simulink model "PulseWidthCalculation"  (R2015b)
settings: Solver=FixedStepDiscrete  StartTime=0.0  StopTime=15  FixedStep=0.01  RelTol=1e-3
undefined symbols (not defined in the file): sigbuilder_block
libraries: simulink x2
settings Model: Creator=MELBAZ1  LastModifiedBy=MELBAZ1

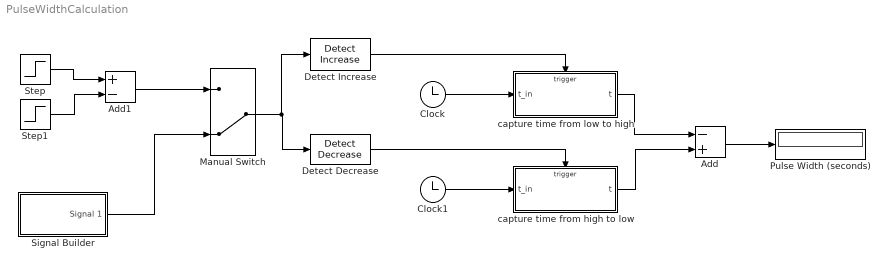
== system PulseWidthCalculation ==
  Add : Sum  Inputs=-+
  Add1 : Sum  Inputs=+-
  Clock : Clock
  Clock1 : Clock
  Detect Decrease : simulink/Logic and Bit Operations/Detect Decrease  vinit=0.0  InputProcessing=Inherited  OutDataTypeStr=boolean
  Detect Increase : simulink/Logic and Bit Operations/Detect Increase  vinit=0.0  InputProcessing=Inherited  OutDataTypeStr=boolean
  Manual Switch : ManualSwitch  CurrentSetting=0
  Pulse Width (seconds) : Display
  Signal Builder : Subsystem  Tag=STV Subsys  LoadFcn=sigbuilder_block('load');  StartFcn=sigbuilder_block('start');  StopFcn=sigbuilder_block('stop');  ClipboardFcn=sigbuilder_block('clipboard');  mask(Sigbuilder block){}
      mask help: Simulink:masks:SigbuilderBlock_MD
      mask init:
      | if ~strcmp(get_param(bdroot(gcbh),'SimulationStatus'),'stopped') tuvar = sigbuilder_block('maskInit'); end
      settings: CopyFcn=sigbuilder_block('copy');  DeleteFcn=sigbuilder_block('delete');  ModelCloseFcn=sigbuilder_block('modelClose');  PreSaveFcn=sigbuilder_block('preSave');  PauseFcn=sigbuilder_block('pause');  ContinueFcn=sigbuilder_block('continue');  NameChangeFcn=sigbuilder_block('namechange');  OpenFcn=sigbuilder_block('open',[453.6 124.2 550.8 400.2 ]);  CloseFcn=sigbuilder_block('close');
      mask Display: plot(0, 0, 100, 100,[2, 2, 32, 32, 2], [68, 8, 8, 68, 68],[32, 2], [38, 38], [32, 19, 2],[53, 60, 44], [32, 17, 17, 2],[16, 16, 31, 31]);txt = getActiveGroup(gcbh);text(2, 100, txt,'verticalAlignment', 'top');
  Step : Step  SampleTime=0.01
  Step1 : Step  Time=1.5  SampleTime=0.01
  capture time from high to low : Subsystem  TreatAsAtomicUnit=on
  "capture time from low to high " : Subsystem  TreatAsAtomicUnit=on
  wires:
  Detect Increase/1 -> "capture time from low to high "/Trigger
  Clock/1 -> "capture time from low to high "/1(t_in)
  Detect Decrease/1 -> capture time from high to low/Trigger
  "capture time from low to high "/1(t) -> Add/1
  capture time from high to low/1(t) -> Add/2
  Clock1/1 -> capture time from high to low/1(t_in)
  Add/1 -> Pulse Width (seconds)/1
  Step/1 -> Add1/1
  Step1/1 -> Add1/2
  Manual Switch/1 -> Detect Increase/1, Detect Decrease/1
  Add1/1 -> Manual Switch/1
  Signal Builder/1(Signal 1) -> Manual Switch/2

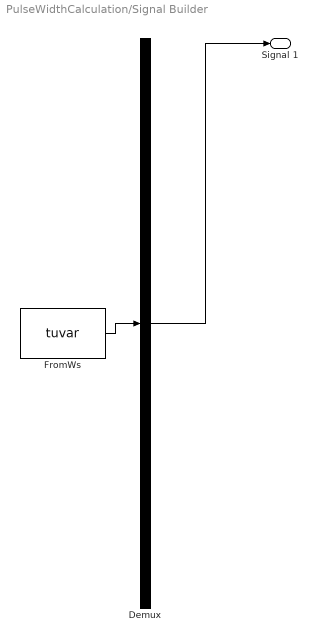
== system PulseWidthCalculation/Signal Builder ==
  Demux : Demux  Tag=STV Demux  Outputs=1
  FromWs : FromWorkspace  Tag=STV FromWs  VariableName=tuvar  SampleTime=0
      SigBuilderData=|
      | common.afterFinalStr = 'Extrapolate'
      | common.sampleTime = 0
      | dataSet.timeRange = [0 10]
      | dataSet.name = 'Group 1'
      | sbobj.Groups.Name = 'Group 1'
      | sbobj.Groups.Signals.Name = 'Signal 1'
      | sbobj.Groups.Signals.XData = [0 4 4 6 6 10]
      | sbobj.Groups.Signals.YData = [0 0 1 1 0 0]
  Signal 1 : Outport  Tag=STV Outport
  wires:
  Demux/1 -> Signal 1/1
  FromWs/1 -> Demux/1

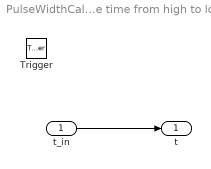
== system PulseWidthCalculation/capture time from high to low ==
  t_in : Inport
  Trigger : TriggerPort
  t : Outport
  wires:
  t_in/1 -> t/1

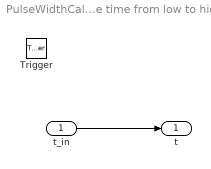
== system PulseWidthCalculation/capture time from low to high  ==
  t_in : Inport
  Trigger : TriggerPort
  t : Outport
  wires:
  t_in/1 -> t/1
